simulink model "harness"  (R2021b)
settings: Solver=VariableStepAuto  StartTime=0.0  StopTime=inf  RelTol=1e-3
libraries: simulink x1
settings Model: Creator=antonio  LastModifiedBy=anton

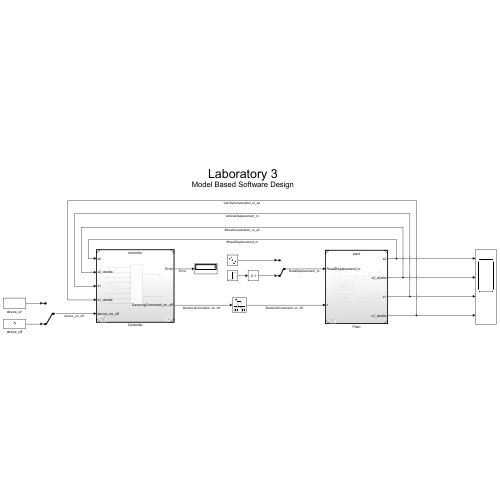
[thumbnail: Simulink's stored preview of the top-level diagram]
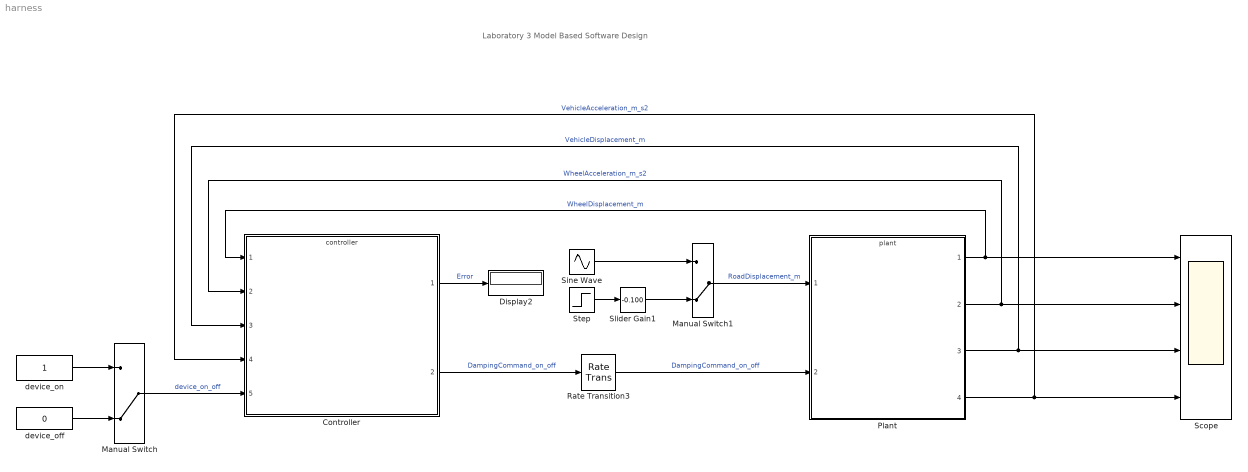
== system harness ==
  note: Laboratory 3
      | Model Based Software Design
  Controller : ModelReference  ModelNameDialog=controller.slx  SimulationMode=Normal  ModelReferenceVersion=1.209
  Display2 : Display
  Manual Switch : ManualSwitch  CurrentSetting=0
  Manual Switch1 : ManualSwitch  CurrentSetting=0
  Plant : ModelReference  ModelNameDialog=plant.slx  SimulationMode=Normal  ModelReferenceVersion=1.30
  Rate Transition3 : RateTransition
  Scope : Scope  NumInputPorts=4
  Sine Wave : Sin  Amplitude=0.05  Frequency=10  SampleTime=0
  Slider Gain1 : simulink/Math Operations/Slider Gain  gain=-0.100  low=-0.2  high=0.2
  Step : Step  Time=0.01  SampleTime=0
  device_off : Constant  Value=0  OutDataTypeStr=int8
  device_on : Constant  OutDataTypeStr=int8
  wires:
  Controller/1 -> Display2/1  "Error"
  Rate Transition3/1 -> Plant/2  "DampingCommand_on_off"
  Step/1 -> Slider Gain1/1
  Plant/3 -> Scope/3, Controller/3  "VehicleDisplacement_m"
  Plant/1 -> Scope/1, Controller/1  "WheelDisplacement_m"
  Plant/2 -> Scope/2, Controller/2  "WheelAcceleration_m_s2"
  Manual Switch1/1 -> Plant/1  "RoadDisplacement_m"
  Slider Gain1/1 -> Manual Switch1/2
  device_on/1 -> Manual Switch/1
  device_off/1 -> Manual Switch/2
  Plant/4 -> Scope/4, Controller/4  "VehicleAcceleration_m_s2"
  Manual Switch/1 -> Controller/5  "device_on_off"
  Sine Wave/1 -> Manual Switch1/1
  Controller/2 -> Rate Transition3/1  "DampingCommand_on_off"
